simulink subsystem "wheelSpeed"  (R2022b)
settings: Solver=VariableStepAuto  StartTime=0.0  StopTime=10.0  RelTol=1e-3
libraries: wheels x4
settings Model: Creator=serga  LastModifiedBy=serga

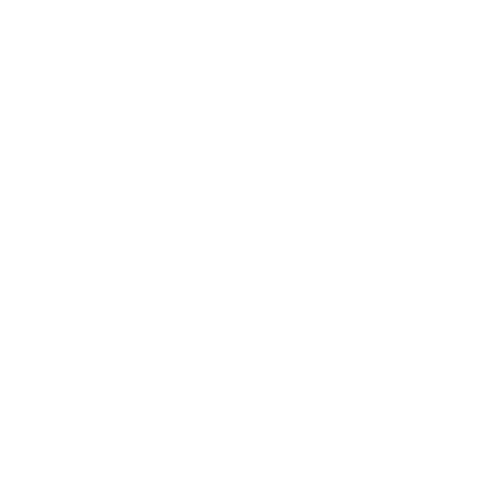
[thumbnail: Simulink's stored preview of the top-level diagram]
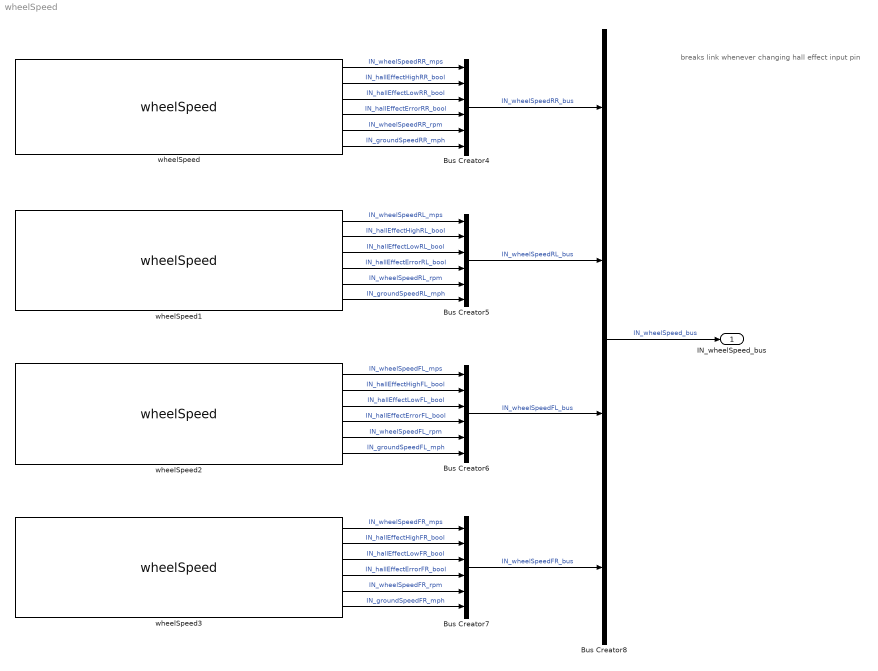
== system wheelSpeed ==
  note: breaks link whenever changing hall effect input pin
  Bus Creator{4..7} (4 alike) : BusCreator  Inputs=6
  Bus Creator8 : BusCreator  Inputs=4
  wheelSpeed : wheels/wheelSpeed  pos='RR'
  wheelSpeed1 : wheels/wheelSpeed  pos='RL'
  wheelSpeed2 : wheels/wheelSpeed  pos='FL'
  wheelSpeed3 : wheels/wheelSpeed  pos='FR'
  IN_wheelSpeed_bus : Outport
  wires:
  wheelSpeed/2 -> Bus Creator4/2  "IN_hallEffectHighRR_bool"
  wheelSpeed3/1 -> Bus Creator7/1  "IN_wheelSpeedFR_mps"
  Bus Creator4/1 -> Bus Creator8/1  "IN_wheelSpeedRR_bus"
  wheelSpeed/6 -> Bus Creator4/6  "IN_groundSpeedRR_mph"
  wheelSpeed2/4 -> Bus Creator6/4  "IN_hallEffectErrorFL_bool"
  wheelSpeed3/4 -> Bus Creator7/4  "IN_hallEffectErrorFR_bool"
  wheelSpeed1/6 -> Bus Creator5/6  "IN_groundSpeedRL_mph"
  wheelSpeed2/6 -> Bus Creator6/6  "IN_groundSpeedFL_mph"
  wheelSpeed/4 -> Bus Creator4/4  "IN_hallEffectErrorRR_bool"
  Bus Creator7/1 -> Bus Creator8/4  "IN_wheelSpeedFR_bus"
  wheelSpeed/3 -> Bus Creator4/3  "IN_hallEffectLowRR_bool"
  wheelSpeed3/5 -> Bus Creator7/5  "IN_wheelSpeedFR_rpm"
  wheelSpeed1/4 -> Bus Creator5/4  "IN_hallEffectErrorRL_bool"
  wheelSpeed2/2 -> Bus Creator6/2  "IN_hallEffectHighFL_bool"
  Bus Creator8/1 -> IN_wheelSpeed_bus/1  "IN_wheelSpeed_bus"
  wheelSpeed1/5 -> Bus Creator5/5  "IN_wheelSpeedRL_rpm"
  wheelSpeed2/1 -> Bus Creator6/1  "IN_wheelSpeedFL_mps"
  wheelSpeed2/3 -> Bus Creator6/3  "IN_hallEffectLowFL_bool"
  wheelSpeed3/6 -> Bus Creator7/6  "IN_groundSpeedFR_mph"
  wheelSpeed3/2 -> Bus Creator7/2  "IN_hallEffectHighFR_bool"
  Bus Creator5/1 -> Bus Creator8/2  "IN_wheelSpeedRL_bus"
  wheelSpeed/5 -> Bus Creator4/5  "IN_wheelSpeedRR_rpm"
  wheelSpeed1/1 -> Bus Creator5/1  "IN_wheelSpeedRL_mps"
  Bus Creator6/1 -> Bus Creator8/3  "IN_wheelSpeedFL_bus"
  wheelSpeed/1 -> Bus Creator4/1  "IN_wheelSpeedRR_mps"
  wheelSpeed3/3 -> Bus Creator7/3  "IN_hallEffectLowFR_bool"
  wheelSpeed1/2 -> Bus Creator5/2  "IN_hallEffectHighRL_bool"
  wheelSpeed2/5 -> Bus Creator6/5  "IN_wheelSpeedFL_rpm"
  wheelSpeed1/3 -> Bus Creator5/3  "IN_hallEffectLowRL_bool"
